simulink model "task2"  (R2021a)
settings: Solver=VariableStepAuto  StartTime=0.0  StopTime=100  RelTol=1e-3
libraries: simulink_extras x4
settings Model: Creator=emiwi425  LastModifiedBy=emiwi425

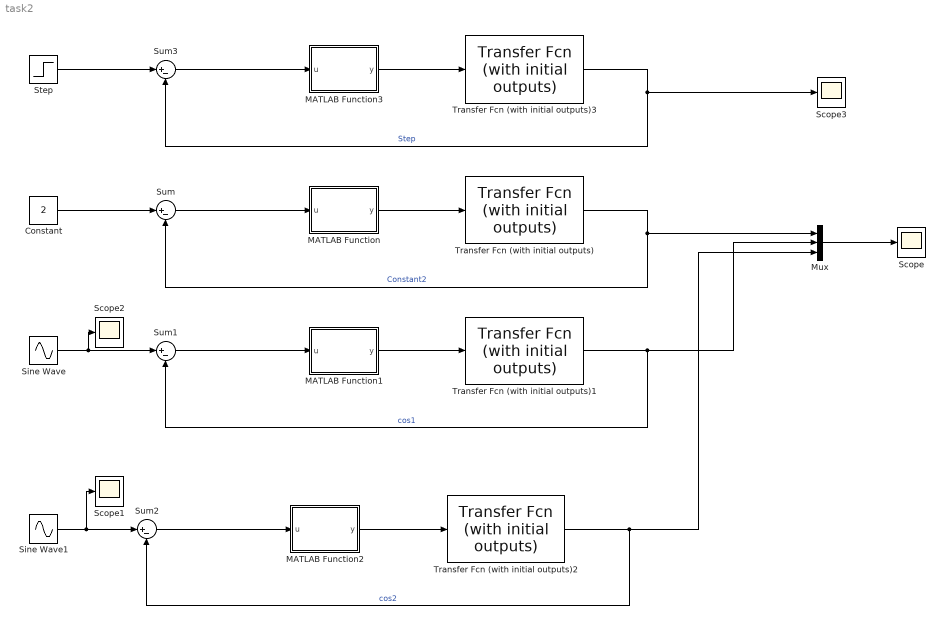
== system task2 ==
  Constant : Constant  Value=2
  MATLAB Function : MATLAB Function  TreatAsAtomicUnit=on
  MATLAB Function1 : MATLAB Function  TreatAsAtomicUnit=on
  MATLAB Function2 : MATLAB Function  TreatAsAtomicUnit=on
  MATLAB Function3 : MATLAB Function  TreatAsAtomicUnit=on
  Mux : Mux  Inputs=3
  Scope{,1..3} (4 alike) : Scope
  Sine Wave : Sin  Amplitude=1/2  Frequency=100  Phase=pi/2  SampleTime=0
  Sine Wave1 : Sin  Amplitude=1/2  Bias=2  Frequency=100  Phase=pi/2  SampleTime=0
  Step : Step  SampleTime=0
  Sum{,1..3} (4 alike) : Sum  Inputs=|+-
  Transfer Fcn (with initial outputs){,1..3} (4 alike) : simulink_extras/Additional Linear/Transfer Fcn (with initial outputs)  N=[1]  D=[1 3 2 0]  Y0=0  U0=0
  wires:
  Sum/1 -> MATLAB Function/1(u)
  MATLAB Function/1(y) -> Transfer Fcn (with initial outputs)/1
  Transfer Fcn (with initial outputs)/1 -> Mux/1, Sum/2  "Constant2"
  Constant/1 -> Sum/1
  Sine Wave/1 -> Scope2/1, Sum1/1
  Sum1/1 -> MATLAB Function1/1(u)
  Transfer Fcn (with initial outputs)1/1 -> Mux/2, Sum1/2  "cos1"
  MATLAB Function1/1(y) -> Transfer Fcn (with initial outputs)1/1
  Sine Wave1/1 -> Scope1/1, Sum2/1
  Sum2/1 -> MATLAB Function2/1(u)
  Transfer Fcn (with initial outputs)2/1 -> Mux/3, Sum2/2  "cos2"
  MATLAB Function2/1(y) -> Transfer Fcn (with initial outputs)2/1
  Mux/1 -> Scope/1
  Sum3/1 -> MATLAB Function3/1(u)
  Transfer Fcn (with initial outputs)3/1 -> Scope3/1, Sum3/2  "Step"
  Step/1 -> Sum3/1
  MATLAB Function3/1(y) -> Transfer Fcn (with initial outputs)3/1

== matlab function task2/MATLAB Function ==
  data: u input; y output
function y = fcn(u)

y = u^3;

== matlab function task2/MATLAB Function2 ==
  data: u input; y output
function y = fcn(u)

y = u^3;

== matlab function task2/MATLAB Function3 ==
  data: u input; y output
function y = fcn(u)

y = u^3;

== matlab function task2/MATLAB Function1 ==
  data: u input; y output
function y = fcn(u)

y = u^3;
